simulink model "ADRC_TD"  (R2022b)
settings: Solver=VariableStepAuto  StartTime=0.0  StopTime=10.0  RelTol=1e-3
model workspace (MAT data in the model file):
  h = 0.01
  h0 = 0.01
  r0 = 1
settings Model: Creator=12854  LastModifiedBy=12854

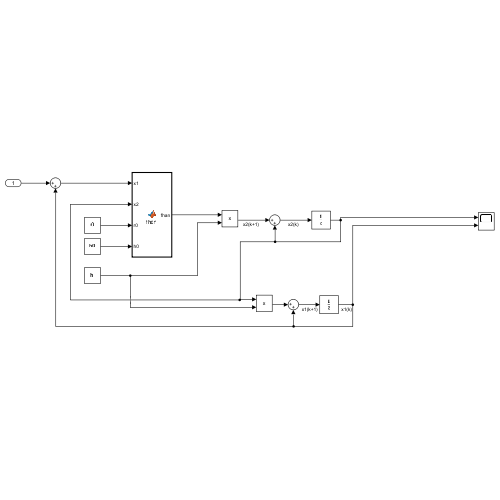
[thumbnail: Simulink's stored preview of the top-level diagram]
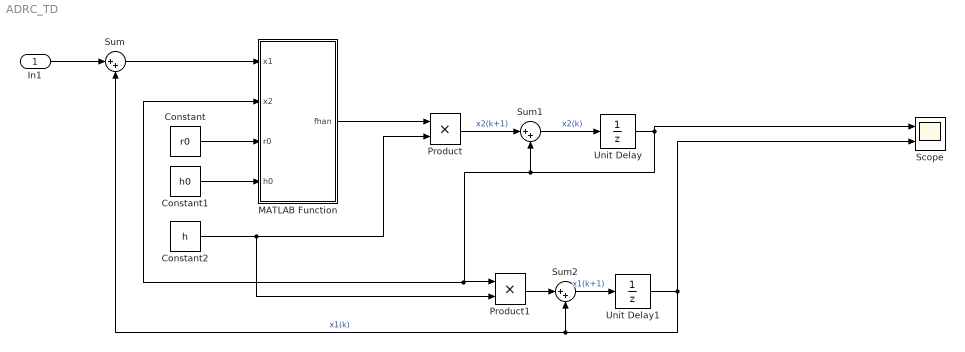
== system ADRC_TD ==
  In1 : Inport
  Constant : Constant  Value=r0
  Constant1 : Constant  Value=h0
  Constant2 : Constant  Value=h
  MATLAB Function : MATLAB Function  TreatAsAtomicUnit=on
  Product : Product
  Product1 : Product
  Scope : Scope  NumInputPorts=2
  Sum : Sum  Inputs=|++
  Sum1 : Sum  Inputs=|++
  Sum2 : Sum  Inputs=|++
  Unit Delay : UnitDelay  SampleTime=-1  HasFrameUpgradeWarning=on
  Unit Delay1 : UnitDelay  SampleTime=-1  HasFrameUpgradeWarning=on
  wires:
  In1/1 -> Sum/1
  Sum/1 -> MATLAB Function/1(x1)
  Constant/1 -> MATLAB Function/3(r0)
  Constant1/1 -> MATLAB Function/4(h0)
  MATLAB Function/1(fhan) -> Product/1
  Constant2/1 -> Product1/2, Product/2
  Product/1 -> Sum1/1  "x2(k+1)"
  Sum1/1 -> Unit Delay/1  "x2(k)"
  Unit Delay/1 -> Scope/1, Product1/1, MATLAB Function/2(x2), Sum1/2
  Product1/1 -> Sum2/1
  Sum2/1 -> Unit Delay1/1  "x1(k+1)"
  Unit Delay1/1 -> Scope/2, Sum2/2, Sum/2  "x1(k)"

== matlab function ADRC_TD/MATLAB Function ==
  data: x1 input; fhan output; x2 input; r0 input; h0 input
% ADRC中的fhan函数（最速综合函数，TD、NLSEF使用）
function fhan = fhan(x1,x2,r0,h0)
d = r0 * (h0^2);
a0 = h0 * x2;
y = x1 + a0;
a1 = sqrt(d * (d + 8 * abs(y)));
a2 = a0 + sign(y) * (a1 - d)/2;
sy = (sign(y + d) - sign(y - d))/2;
a = (a0 + y - a2) * sy + a2;
sa = (sign(a + d) - sign(a - d))/2;
fhan = -r0 * (a / d - sign(a)) * sa - r0 * sign(a);
